simulink model "Model"  (R2021b)
settings: Solver=VariableStepAuto  StartTime=0.0  StopTime=SimTime  FixedStep=1  RelTol=1e-13  AbsTol=1e-13
values from neighbouring files (symbols this model uses):
  a = (39376)*1e3    (= 39376000)    [ScriptGroup20.m]
  alphaxy = (alphaxy/3)^2    (= 2.60887104e-10)    [ScriptGroup20.m]
  alphaz = (alphaz/3)^2    (= 3.75687767111e-08)    [ScriptGroup20.m]
  Aorthsens = 1e-3.*[1000,0.2,0.2;0.2,1000,0.2;0.2,0.2,1000]    [ScriptGroup20.m]
  burn_angle = deg2rad(30)    [ScriptGroup20.m]
  Controlled = 1    [ScriptGroup20.m]
  e = 0.7596    [ScriptGroup20.m]
  fgyro = 5    [ScriptGroup20.m]
  Fmax = 0.325/2    (= 0.1625)    [ScriptGroup20.m]
  fst = 5    [ScriptGroup20.m]
  hr0 = hrwslew(:,end)    [ScriptGroup20.m]
  i = deg2rad(28.4252)    [ScriptGroup20.m]
  I_tensor = I_unpacked    [ScriptGroup20.m]
  Iinv_tensor = inv(I_tensor)    [ScriptGroup20.m]
  Kdtrack = Kdtrack_track    (= 0.009)    [ScriptGroup20.m]
  Kpdet = 0.3    [ScriptGroup20.m]
  Kptrack = Kptrack_track    (= 0.009)    [ScriptGroup20.m]
  m_sc = factor*[1;1;1]    [ScriptGroup20.m]
  maxH = 50*1e-3    (= 0.05)    [ScriptGroup20.m]
  maxT = 8*1e-3    (= 0.008)    [ScriptGroup20.m]
  ModCont = 1    [ScriptGroup20.m]
  mu = 3.98600433e+5*1e9    (= 398600433000000)    [ScriptGroup20.m]
  normals = [n1,n2,n3,n4,n5,n6,n7,n8,n9,n10]    [ScriptGroup20.m]
  omega = deg2rad(0)    [ScriptGroup20.m]
  phi0 = Angtrueslew(1,1,end)    [ScriptGroup20.m]
  propmat = [rhos_sc;rhod_sc;rhos_sp;rhod_sp]    [ScriptGroup20.m]
  propsurf = [A1,A2,A3,A1,A2,A3,A7,A7,A9,A9]    [ScriptGroup20.m]
  psi0 = Angtrueslew(3,1,end)    [ScriptGroup20.m]
  r_cpTocm = [r1,r2,r3,r4,r5,r6,r7,r8,r9,r10]-ones(3,10).*cm    [ScriptGroup20.m]
  Re = 6371.01*1e3    (= 6371010)    [ScriptGroup20.m]
  sigma = deg2rad(0)    [ScriptGroup20.m]
  starcat = zeros(height(starcattab)-2,2)    [ScriptGroup20.m]
  T = R2*R1*[x*sin(gamma),-x*sin(gamma),x*sin(gamma),-x*sin(gamma);         -x*cos(gamma),l*sin(gamma),x*cos(gamma),-l*sin(gamma);         -l*sin(gamma),x*cos(gamma),l*sin(gamma),-x*cos(gamma)]    [ScriptGroup20.m]
  theta0 = Angtrueslew(2,1,end)    [ScriptGroup20.m]
  theta0orb = forbitslew(end)    [ScriptGroup20.m]
  thetb = thetb^2    [ScriptGroup20.m]
  thetn = thetn^2    [ScriptGroup20.m]
  thetsperc = 5*1e-4    (= 0.0005)    [ScriptGroup20.m]
  w = null(T)    [ScriptGroup20.m]
  w0_vector = wgyroslew(:,1,end)    [ScriptGroup20.m]
  w_lim = deg2rad(3)    [ScriptGroup20.m]
undefined symbols (not defined in the file or in its folder): DiscIntNeverNeededParam, phi_0, psi_0, theta_0
libraries: dspindex x22, matrix_library x20, vrlib x6, dspinverses x3, simulink_extras x3, dspfdesign x3, dspmtrx3 x2, simulink x1
(part 1 of 2)
settings Model: Creator=giova  LastModifiedBy=giova
settings SolverCC: ZeroCrossAlgorithm=Adaptive
settings OptimizationCC: BlockReduction=off  DefaultParameterBehavior=Inlined  BufferReuse=off
settings DebuggingCC: IgnoredZcDiagnostic=none

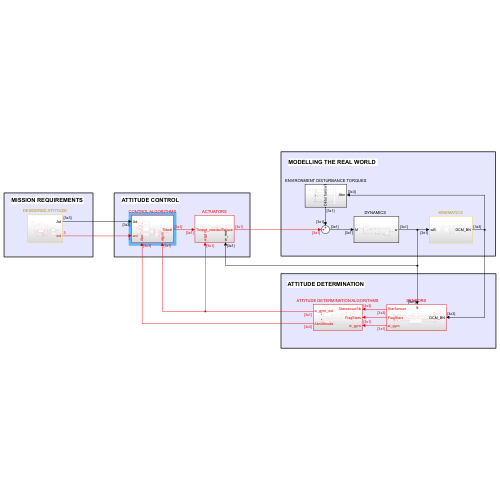
[thumbnail: Simulink's stored preview of the top-level diagram]
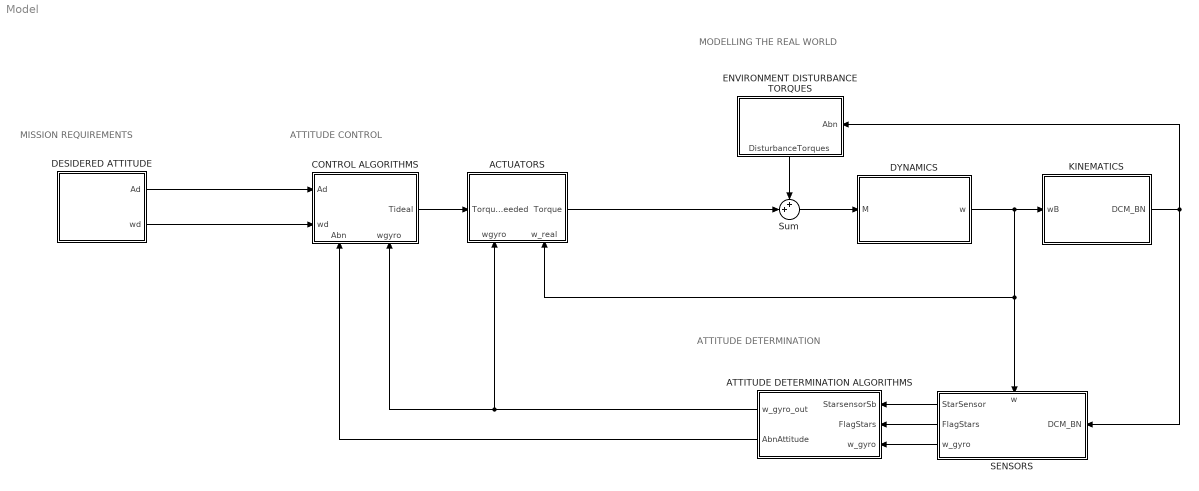
== system Model ==
  note: MODELLING THE REAL WORLD
  note: ATTITUDE DETERMINATION
  note: MISSION REQUIREMENTS
  note: ATTITUDE CONTROL
  ACTUATORS : Subsystem
      settings: PortSchema="{\"entries\":[{\"content\":{\"sides\":[{\"content\":{\"connectorIds\":[\"In1\"]},\"type\":\"ConnectorPlacement.EquallySpacedRectSide\",\"uuid\":\"28bcfce0-0d34-469d-9776-74cc58e318fa\"},{\"content\":{\"connectorIds\":[\"Out1\"],\"side\":\"RIGHT\"},\"type\":\"ConnectorPlacement.EquallySpacedRectSide\",\"uuid\":\"2255c173-df7a-4664-85cc-96c785adaea5\"},{\"content\":{\"connectorIds\":[],\"side\":\"TOP\"},\"type\":\"ConnectorPlacement.EquallySpacedRectSide\",\"uuid\":\"32c912d7-9334-4d54-9f32-8ee23b9abac0\"},{\"content\":{\"connectorIds\":[\"In2\",\"In3\"],\"side\":\"BOTTOM\"},\"type\":\"ConnectorPlacement.EquallySpacedRectSide\",\"uuid\":\"2cb89a57-816b-4867-95bb-5d60911795f4\"}]},\"type\":\"ConnectorPlacement.EquallySpacedConnector\",\"uuid\":\"77867389-a468-4a3c-acb5-d08783c7db16\"}],\"packageUris\":[\"http://schema.mathworks.com/mf0/Connector/R2020b\"],\"version\":\"1.0\"}"
  ATTITUDE DETERMINATION ALGORITHMS : Subsystem
  CONTROL ALGORITHMS : Subsystem
      settings: PortSchema="{\"entries\":[{\"content\":{\"sides\":[{\"content\":{\"connectorIds\":[\"In1\",\"In2\"]},\"type\":\"ConnectorPlacement.EquallySpacedRectSide\",\"uuid\":\"73dddf99-4801-43df-975c-c163be84342b\"},{\"content\":{\"connectorIds\":[\"Out1\"],\"side\":\"RIGHT\"},\"type\":\"ConnectorPlacement.EquallySpacedRectSide\",\"uuid\":\"0da970fe-52f5-407f-b1e9-9d4b0160e11a\"},{\"content\":{\"connectorIds\":[],\"side\":\"TOP\"},\"type\":\"ConnectorPlacement.EquallySpacedRectSide\",\"uuid\":\"7ba04c9a-5ad7-470a-a631-d233976ad8b8\"},{\"content\":{\"connectorIds\":[\"In3\",\"In4\"],\"side\":\"BOTTOM\"},\"type\":\"ConnectorPlacement.EquallySpacedRectSide\",\"uuid\":\"5f2d3d06-e891-478c-9602-3776d7c735db\"}]},\"type\":\"ConnectorPlacement.EquallySpacedConnector\",\"uuid\":\"a8e1a751-f603-45b5-97f1-265969e24c76\"}],\"packageUris\":[\"http://schema.mathworks.com/mf0/Connector/R2020b\"],\"version\":\"1.0\"}"
  DESIDERED ATTITUDE : Subsystem
  "DYNAMICS  " : Subsystem
  ENVIRONMENT DISTURBANCE TORQUES : Subsystem
      settings: PortSchema="{\"entries\":[{\"content\":{\"sides\":[{\"content\":{\"connectorIds\":[\"In1\"]},\"type\":\"ConnectorPlacement.EquallySpacedRectSide\",\"uuid\":\"a2be9383-99de-4e0f-aff6-078514624980\"},{\"content\":{\"connectorIds\":[],\"side\":\"RIGHT\"},\"type\":\"ConnectorPlacement.EquallySpacedRectSide\",\"uuid\":\"8c8f0942-4a2a-4cb8-b252-92284a086b4d\"},{\"content\":{\"connectorIds\":[\"Out1\"],\"side\":\"TOP\"},\"type\":\"ConnectorPlacement.EquallySpacedRectSide\",\"uuid\":\"b1ad7016-209b-4a42-9402-dc7624b55aba\"}]},\"type\":\"ConnectorPlacement.EquallySpacedConnector\",\"uuid\":\"7a786cca-b338-4110-b1b1-81221cfdfe5d\"}],\"packageUris\":[\"http://schema.mathworks.com/mf0/Connector/R2020b\"],\"version\":\"1.0\"}"
  KINEMATICS : Subsystem
  SENSORS : Subsystem
      settings: PortSchema="{\"entries\":[{\"content\":{\"sides\":[{\"content\":{\"connectorIds\":[\"In1\"]},\"type\":\"ConnectorPlacement.EquallySpacedRectSide\",\"uuid\":\"b510f6ef-f21e-411c-8ea4-8a9ce0e96801\"},{\"content\":{\"connectorIds\":[\"Out1\",\"Out2\",\"Out3\"],\"side\":\"RIGHT\"},\"type\":\"ConnectorPlacement.EquallySpacedRectSide\",\"uuid\":\"2c17a393-d83e-490b-b8d9-3edd4b192ceb\"},{\"content\":{\"connectorIds\":[],\"side\":\"TOP\"},\"type\":\"ConnectorPlacement.EquallySpacedRectSide\",\"uuid\":\"72c4e30b-e03c-45bc-abfe-ce46fe4af89d\"},{\"content\":{\"connectorIds\":[\"In2\"],\"side\":\"BOTTOM\"},\"type\":\"ConnectorPlacement.EquallySpacedRectSide\",\"uuid\":\"41e20ae9-4ca7-4038-b613-5a3bc8a297c6\"}]},\"type\":\"ConnectorPlacement.EquallySpacedConnector\",\"uuid\":\"248ff9f1-2acb-4da2-b04a-a2681fb74a40\"}],\"packageUris\":[\"http://schema.mathworks.com/mf0/Connector/R2020b\"],\"version\":\"1.0\"}"
  Sum : Sum  Inputs=++|
  wires:
  KINEMATICS/1(DCM_BN) -> SENSORS/1(DCM_BN), ENVIRONMENT DISTURBANCE TORQUES/1(Abn)
  "DYNAMICS  "/1(w) -> KINEMATICS/1(wB), ACTUATORS/3(w_real), SENSORS/2(w)
  Sum/1 -> "DYNAMICS  "/1(M)
  ENVIRONMENT DISTURBANCE TORQUES/1(DisturbanceTorques) -> Sum/1
  SENSORS/2(FlagStars) -> ATTITUDE DETERMINATION ALGORITHMS/2(FlagStars)
  SENSORS/3(StarSensor) -> ATTITUDE DETERMINATION ALGORITHMS/1(StarsensorSb)
  SENSORS/1(w_gyro) -> ATTITUDE DETERMINATION ALGORITHMS/3(w_gyro)
  ACTUATORS/1(Torque) -> Sum/2
  DESIDERED ATTITUDE/1(Ad) -> CONTROL ALGORITHMS/1(Ad)
  ATTITUDE DETERMINATION ALGORITHMS/1(w_gyro_out) -> CONTROL ALGORITHMS/4(wgyro), ACTUATORS/2(wgyro)
  ATTITUDE DETERMINATION ALGORITHMS/2(AbnAttitude) -> CONTROL ALGORITHMS/3(Abn)
  CONTROL ALGORITHMS/1(Tideal) -> ACTUATORS/1(Torque_needed)
  DESIDERED ATTITUDE/2(wd) -> CONTROL ALGORITHMS/2(wd)

== system Model/ACTUATORS ==
  Torque_needed : Inport
  wgyro : Inport  Port=2
  w_real : Inport  Port=3
  Constant : Constant  Value=[0;0;0]
  RW : Subsystem
  Sum : Sum
  Switch : Switch  Criteria=u2 > Threshold
  Thruster : Subsystem
  To Workspace : ToWorkspace  VariableName=simout7  SaveFormat=Timeseries  SampleTime=-1
  To Workspace1 : ToWorkspace  VariableName=simout9  SaveFormat=Timeseries  SampleTime=-1
  Torque : Outport
  wires:
  Sum/1 -> To Workspace/1, Torque/1
  wgyro/1 -> RW/2(wgyro)
  RW/2(Treal) -> Sum/2
  Thruster/1(TorqueReal) -> Switch/1
  Constant/1 -> Switch/3
  Switch/1 -> To Workspace1/1, Sum/1
  Torque_needed/1 -> RW/1(Torque_needed), Thruster/1(Torqueneeded)
  RW/1(FlagDesat) -> Switch/2
  w_real/1 -> RW/3(w_real)

== system Model/ATTITUDE DETERMINATION ALGORITHMS ==
  StarsensorSb : Inport
  FlagStars : Inport  Port=2
  w_gyro : Inport  Port=3
  Kinematics with update from Star Tracker1 : Subsystem
  Switch : Switch  Criteria=u2 ~= 0
  SwitchAttitudeDetermination : Subsystem
  To Workspace : ToWorkspace  VariableName=simout1  SaveFormat=Timeseries  SampleTime=-1
  w_gyro_out : Outport
  AbnAttitude : Outport  Port=2
  wires:
  Kinematics with update from Star Tracker1/1(DCM_BN_gyro) -> Switch/3
  SwitchAttitudeDetermination/1(star_out) -> Kinematics with update from Star Tracker1/3(star_out), Switch/2
  FlagStars/1 -> SwitchAttitudeDetermination/2(FlagStars)
  StarsensorSb/1 -> Switch/1, Kinematics with update from Star Tracker1/1(DCM_BN_star)
  Switch/1 -> AbnAttitude/1, To Workspace/1, SwitchAttitudeDetermination/3(Abnsensors)
  w_gyro/1 -> SwitchAttitudeDetermination/1(wB_m), w_gyro_out/1, Kinematics with update from Star Tracker1/2(wB_m)

== system Model/CONTROL ALGORITHMS ==
  Ad : Inport
  wd : Inport  Port=2
  Abn : Inport  Port=3
  wgyro : Inport  Port=4
  Constant : Constant  Value=ModCont
  Constant1 : Constant  Value=[0;0;0]
  Constant2 : Constant  Value=Controlled
  De-tumbling : Subsystem
  Pointing error : Subsystem
      settings: PortSchema="{\"entries\":[{\"content\":{\"sides\":[{\"content\":{\"connectorIds\":[]},\"type\":\"ConnectorPlacement.EquallySpacedRectSide\",\"uuid\":\"59077e71-7c09-4a90-bf3b-715fb2f3e64a\"},{\"content\":{\"connectorIds\":[\"In1\",\"In2\"],\"side\":\"RIGHT\"},\"type\":\"ConnectorPlacement.EquallySpacedRectSide\",\"uuid\":\"5359064d-45c1-447c-a242-520af2c8ee16\"},{\"content\":{\"connectorIds\":[],\"side\":\"TOP\"},\"type\":\"ConnectorPlacement.EquallySpacedRectSide\",\"uuid\":\"50cd8bf9-1849-445b-b3a9-8b2cd9485115\"}]},\"type\":\"ConnectorPlacement.EquallySpacedConnector\",\"uuid\":\"6167e8e7-e0c2-4106-8eb9-df9ff1faf5b0\"}],\"packageUris\":[\"http://schema.mathworks.com/mf0/Connector/R2020b\"],\"version\":\"1.0\"}"
  Switch : Switch  Criteria=u2 > Threshold
  Switch1 : Switch  Criteria=u2 > Threshold
  Tracking : Subsystem
  Tideal : Outport
  wires:
  Abn/1 -> Tracking/2(Abn), Pointing error/2(Abnsen)
  Ad/1 -> Tracking/1(Ad), Pointing error/1(Ad)
  wgyro/1 -> Tracking/4(wgyro), De-tumbling/1(w)
  De-tumbling/1(Tdet) -> Switch/3
  Constant/1 -> Switch/2
  Constant1/1 -> Switch1/3
  Constant2/1 -> Switch1/2
  Tracking/1(Ttrack) -> Switch/1
  Switch/1 -> Switch1/1
  Switch1/1 -> Tideal/1
  wd/1 -> Tracking/3(wd)

== system Model/DESIDERED ATTITUDE ==
  Constant : Constant  Value=sigma
  Constant1 : Constant  Value=i
  Constant2 : Constant  Value=omega
  Constant3 : Constant  Value=a
  Constant4 : Constant  Value=e
  Constant5 : Constant  Value=0
  Discrete-Time Integrator : DiscreteIntegrator  InitialCondition=theta0orb  SampleTime=-1  ICPrevOutput=DiscIntNeverNeededParam  ICPrevScaledInput=DiscIntNeverNeededParam
  From N to eph : MATLAB Function  TreatAsAtomicUnit=on
  From eph to rthetah : MATLAB Function  TreatAsAtomicUnit=on
  Mux : Mux  Inputs=3
  Subsystem1 : Subsystem
  To Workspace : ToWorkspace  VariableName=simout8  SaveFormat=Timeseries  SampleTime=-1
  Ad : Outport
  wd : Outport  Port=2
  wires:
  Constant/1 -> From N to eph/1(sigma)
  Constant1/1 -> From N to eph/2(i)
  Constant2/1 -> From N to eph/3(omega)
  Discrete-Time Integrator/1 -> To Workspace/1, From eph to rthetah/2(theta), Subsystem1/3(Theta)  "theta"
  Constant4/1 -> Subsystem1/1(e)
  Constant3/1 -> Subsystem1/2(a)
  From N to eph/1(Aeph) -> From eph to rthetah/1(Aeph)
  From eph to rthetah/1(Arthetah) -> Ad/1
  Subsystem1/1(ThetaDot) -> Mux/3, Discrete-Time Integrator/1
  Constant5/1 -> Mux/1, Mux/2
  Mux/1 -> wd/1

== system Model/DYNAMICS   ==
  M : Inport
  Constant : Constant  Value=I_tensor
  Constant1 : Constant  Value=Iinv_tensor
  Cross Product : vrlib/Utilities/Cross Product
  Integrator : Integrator  InitialCondition=w0_vector
  Product : Product  Multiplication=Matrix(*)
  Product1 : Product  Multiplication=Matrix(*)
  Sum : Sum  Inputs=+-
  w : Outport
  wires:
  Constant1/1 -> Product1/1
  Sum/1 -> Product1/2  "w'"
  Product1/1 -> Integrator/1
  Cross Product/1 -> Sum/2
  M/1 -> Sum/1
  Constant/1 -> Product/1
  Product/1 -> Cross Product/2
  Integrator/1 -> w/1, Product/2, Cross Product/1  "w"

== system Model/ENVIRONMENT DISTURBANCE TORQUES ==
  Abn : Inport
  Gravity Gradient Torque : Subsystem
  MagneticTorque : Subsystem
  OrbitRadialDirection : Subsystem
  Product1 : Product  Multiplication=Matrix(*)
  SRPTorque : Subsystem
  Subsystem : Subsystem
  Sum : Sum  Inputs=+++
  SunPositionRespectN : Subsystem
  To Workspace : ToWorkspace  VariableName=simout6  SaveFormat=Timeseries  SampleTime=-1
  DisturbanceTorques : Outport
  wires:
  Sum/1 -> To Workspace/1, DisturbanceTorques/1
  Gravity Gradient Torque/1(GravityTorque) -> Sum/3
  OrbitRadialDirection/2(Aln) -> Gravity Gradient Torque/2(Aln)
  MagneticTorque/1(MagneticTorque) -> Sum/1
  SunPositionRespectN/1(sn) -> Subsystem/2(rs), Product1/2
  Product1/1 -> SRPTorque/2(sb)  "sb"
  OrbitRadialDirection/1(rn) -> Gravity Gradient Torque/3(rn), Subsystem/1(rn), MagneticTorque/1(rn)
  SRPTorque/1(SRPTorque) -> Sum/2
  Abn/1 -> MagneticTorque/2(Abn), Product1/1, Gravity Gradient Torque/1(Abn)
  Subsystem/1(flag_eclipse) -> SRPTorque/1(SwitchEclipse)

== system Model/KINEMATICS ==
  wB : Inport
  312 Euler Angles : Subsystem
  313 Euler Angles : Subsystem
  Constant : Constant  Value=[phi0;theta0;psi0]
  Delay One Step : Delay  DelayLength=1  InitialConditionSource=Input port
      settings: InputPortMap=u0,p4
  Delay One Step1 : Delay  DelayLength=1  InitialConditionSource=Input port
      settings: InputPortMap=u0,p4
  Factotum Switch : MATLAB Function  TreatAsAtomicUnit=on
  FinalConditions : Subsystem
  Initial condition : MATLAB Function  TreatAsAtomicUnit=on
  Switch : Switch  Criteria=u2 ~= 0
  DCM_BN : Outport
  wires:
  wB/1 -> 313 Euler Angles/1(wB), 312 Euler Angles/3(wB)
  312 Euler Angles/1(DCM_BN_312) -> Switch/1
  313 Euler Angles/1(DCM_BN_313) -> Switch/3
  Factotum Switch/1(IC_312) -> 312 Euler Angles/1(IC_312)
  Factotum Switch/3(IC_313) -> 313 Euler Angles/3(IC_313)
  Switch/1 -> DCM_BN/1, FinalConditions/1(DCM), Delay One Step1/1
  Factotum Switch/2(flagOut) -> Delay One Step/1, 313 Euler Angles/2(flag), Switch/2, 312 Euler Angles/2(flag)
  Delay One Step/1 -> Factotum Switch/2(flagIn)
  Delay One Step1/1 -> Factotum Switch/1(DCM_BN)
  Constant/1 -> Initial condition/1(EA_BN_0)
  Initial condition/2(flagIn_0) -> Delay One Step/2
  Initial condition/1(DCM_BN_0) -> Delay One Step1/2

== system Model/SENSORS ==
  DCM_BN : Inport
  w : Inport  Port=2
  Gyro : Subsystem
  StarCat : Subsystem
  To Workspace : ToWorkspace  VariableName=simout  SaveFormat=Timeseries  SampleTime=-1
  Zero-Order Hold1 : ZeroOrderHold  SampleTime=1/fst
  Zero-Order Hold2 : ZeroOrderHold  SampleTime=1/fst
  w_gyro : Outport
  FlagStars : Outport  Port=2
  StarSensor : Outport  Port=3
  wires:
  DCM_BN/1 -> Zero-Order Hold1/1
  Zero-Order Hold1/1 -> StarCat/1(Abn)
  w/1 -> Zero-Order Hold2/1
  Zero-Order Hold2/1 -> Gyro/1(w)
  Gyro/1(w_gyro) -> To Workspace/1, w_gyro/1
  StarCat/1(StarSensor) -> StarSensor/1
  StarCat/2(FlagStars) -> FlagStars/1

== system Model/ACTUATORS/RW ==
  Torque_needed : Inport
  wgyro : Inport  Port=2
  w_real : Inport  Port=3
  Aconfiguration : Constant  Value=[1,0,0,1/sqrt(3);0,1,0,1/sqrt(3);0,0,1,1/sqrt(3)]  SampleTime=1/fgyro
  Mapping actuator : Subsystem
  RealRW : Subsystem
      settings: PortSchema="{\"entries\":[{\"content\":{\"sides\":[{\"content\":{\"connectorIds\":[\"In1\",\"In2\"]},\"type\":\"ConnectorPlacement.EquallySpacedRectSide\",\"uuid\":\"4cf3556b-d79b-4b35-83c7-165ec12fb347\"},{\"content\":{\"connectorIds\":[\"Out1\",\"Out2\"],\"side\":\"RIGHT\"},\"type\":\"ConnectorPlacement.EquallySpacedRectSide\",\"uuid\":\"b017f686-de2a-46f5-bc21-38e4657d98f2\"},{\"content\":{\"connectorIds\":[\"In3\"],\"side\":\"TOP\"},\"type\":\"ConnectorPlacement.EquallySpacedRectSide\",\"uuid\":\"e19596cf-63b5-4569-a83e-a83db9975230\"}]},\"type\":\"ConnectorPlacement.EquallySpacedConnector\",\"uuid\":\"677db8a5-061d-4d8b-93d2-fe0edb0a0b58\"}],\"packageUris\":[\"http://schema.mathworks.com/mf0/Connector/R2020b\"],\"version\":\"1.0\"}"
  FlagDesat : Outport
  Treal : Outport  Port=2
  wires:
  Torque_needed/1 -> Mapping actuator/1(Uideal)
  wgyro/1 -> Mapping actuator/2(w_gyro)
  Aconfiguration/1 -> RealRW/1(Configuration), Mapping actuator/3(Configuration)
  RealRW/1(Ureal) -> Treal/1
  Mapping actuator/1(ElectricMotor) -> RealRW/3(Mr)
  RealRW/2(FlagDesat) -> FlagDesat/1
  w_real/1 -> RealRW/2(w_real)

== system Model/ACTUATORS/Thruster ==
  Torqueneeded : Inport
  Constant : Constant  Value=T  SampleTime=1/fgyro
  Constant4 : Constant  Value=w
  Divide : Product  Inputs=*/
  Max : MinMax  Function=max
  On/Off logic : Subsystem
  Product : Product  Multiplication=Matrix(*)
  Product1 : Product
  Product2 : Product  Multiplication=Matrix(*)
  Pseudoinverse : dspinverses/Pseudoinverse  wanterr=off  SimulateUsing=Interpreted execution
      settings: SourceProductBaseCode=DS
  Scope : Scope
  Sum : Sum
  TorqueReal : Outport
  wires:
  Constant/1 -> Pseudoinverse/1, Product2/1
  Torqueneeded/1 -> Product/2
  Pseudoinverse/1 -> Product/1
  Product/1 -> Sum/2, Divide/1
  Divide/1 -> Max/1
  Product1/1 -> Sum/1
  Constant4/1 -> Product1/2, Divide/2  "null space"
  Product2/1 -> TorqueReal/1
  On/Off logic/1(Freal) -> Product2/2, Scope/1
  Sum/1 -> On/Off logic/1(Fideal)
  Max/1 -> Product1/1

== system Model/ATTITUDE DETERMINATION ALGORITHMS/Kinematics with update from Star Tracker1 ==
  DCM_BN_star : Inport
  wB_m : Inport  Port=2
  star_out : Inport  Port=3
  312 Euler Angles : Subsystem
  313 Euler Angles : Subsystem
  Delay One Step : Delay  DelayLength=1  InitialConditionSource=Input port
      settings: InputPortMap=u0,p4
  Delay One Step1 : Delay  DelayLength=1  InitialConditionSource=Input port
      settings: InputPortMap=u0,p4
  Factotum Switch : MATLAB Function  TreatAsAtomicUnit=on
  Initial condition : MATLAB Function  TreatAsAtomicUnit=on
  MATLAB Function : MATLAB Function  TreatAsAtomicUnit=on
  MATLAB Function1 : MATLAB Function  TreatAsAtomicUnit=on
  Scope : Scope
  Switch : Switch  Criteria=u2 ~= 0
  DCM_BN_gyro : Outport
  wires:
  Factotum Switch/1(IC_312) -> MATLAB Function/2(IC_312_in)
  Factotum Switch/3(IC_313) -> MATLAB Function1/3(IC_313_in)
  MATLAB Function1/2(IC_313_out) -> 313 Euler Angles/3(IC_313)
  MATLAB Function1/1(flag_out) -> 313 Euler Angles/2(flag)
  star_out/1 -> MATLAB Function1/1(star_out), MATLAB Function/4(star_out)
  MATLAB Function/2(flag_out) -> 312 Euler Angles/2(flag)
  MATLAB Function/1(IC_312_out) -> 312 Euler Angles/1(IC_312)
  Initial condition/1(flagIn_0) -> Delay One Step/2
  DCM_BN_star/1 -> MATLAB Function/1(DCM_BN_star), Delay One Step1/2, MATLAB Function1/4(DCM_BN_star), Initial condition/1(DCM_BN_star)
  Delay One Step1/1 -> Factotum Switch/1(DCM_BN)
  Delay One Step/1 -> Factotum Switch/2(flagIn)
  Factotum Switch/2(flagOut) -> Scope/1, Switch/2, Delay One Step/1, MATLAB Function1/2(flag_in), MATLAB Function/3(flag_in)
  Switch/1 -> Delay One Step1/1, DCM_BN_gyro/1
  313 Euler Angles/1(DCM_BN_313) -> Switch/3
  312 Euler Angles/1(DCM_BN_312) -> Switch/1
  wB_m/1 -> 312 Euler Angles/3(wB), 313 Euler Angles/1(wB)

== system Model/ATTITUDE DETERMINATION ALGORITHMS/SwitchAttitudeDetermination ==
  wB_m : Inport
  FlagStars : Inport  Port=2
  Abnsensors : Inport  Port=3
  Constant : Constant  Value=[0; 0; 1]  VectorParams1D=off
  Constant1 : Constant  Value=burn_angle
  Constant2 : Constant  Value=w_lim
  Delay : Delay  DelayLength=1  InitialCondition=[1,0,0;0,1,0;0,0,1]
  Dot Product : DotProduct  InputSameDT=on  OutDataTypeStr=Inherit: Inherit via internal rule
  MATLAB Function : MATLAB Function  TreatAsAtomicUnit=on
  Product : Product  Multiplication=Matrix(*)
  SunPositionRespectN : Subsystem
  star_out : Outport
  wires:
  SunPositionRespectN/1(sn) -> Product/2
  Constant2/1 -> MATLAB Function/4(w_lim)
  Constant1/1 -> MATLAB Function/3(burn_angle)
  Constant/1 -> Dot Product/2
  FlagStars/1 -> MATLAB Function/5(FlagStars)
  Abnsensors/1 -> Delay/1
  Dot Product/1 -> MATLAB Function/2(cos_alpha)
  wB_m/1 -> MATLAB Function/1(wB_m)
  MATLAB Function/1(star_out) -> star_out/1
  Product/1 -> Dot Product/1
  Delay/1 -> Product/1

== system Model/CONTROL ALGORITHMS/De-tumbling ==
  w : Inport
  Gain : Gain  Gain=-Kpdet
  Tdet : Outport
  wires:
  w/1 -> Gain/1
  Gain/1 -> Tdet/1

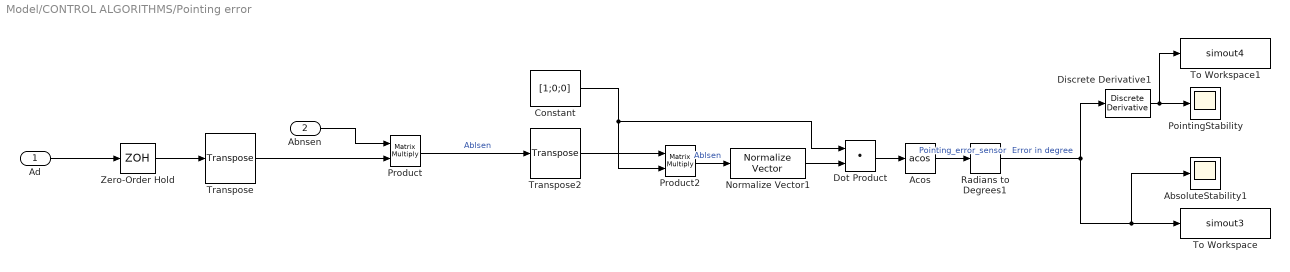
== system Model/CONTROL ALGORITHMS/Pointing error ==
  Ad : Inport
  Abnsen : Inport  Port=2
  AbsoluteStability1 : Scope
  Acos : Trigonometry  Operator=acos
  Constant : Constant  Value=[1;0;0]
  Discrete Derivative1 : simulink/Discrete/Discrete Derivative  gainval=1.0  ICPrevScaledInput=0.0  OutMin=[]  OutMax=[]  OutDataType=fixdt(1, 16)  OutScaling=2^-10  DoSatur=off
  Dot Product : DotProduct  InputSameDT=on  OutDataTypeStr=Inherit: Inherit via internal rule
  Normalize Vector1 : vrlib/Utilities/Normalize Vector  maxzero=0
  PointingStability : Scope
  Product : Product  Multiplication=Matrix(*)
  Product2 : Product  Multiplication=Matrix(*)
  Radians to Degrees1 : simulink_extras/Transformations/Radians to Degrees
  To Workspace : ToWorkspace  VariableName=simout3  SaveFormat=Timeseries  SampleTime=-1
  To Workspace1 : ToWorkspace  VariableName=simout4  SaveFormat=Timeseries  SampleTime=-1
  Transpose : matrix_library/Transpose
      settings: SourceProductBaseCode=SL
  Transpose2 : matrix_library/Transpose
      settings: SourceProductBaseCode=SL
  Zero-Order Hold : ZeroOrderHold  SampleTime=1/fgyro
  wires:
  Ad/1 -> Zero-Order Hold/1
  Zero-Order Hold/1 -> Transpose/1
  Product/1 -> Transpose2/1  "Ablsen"
  Transpose/1 -> Product/2
  Abnsen/1 -> Product/1
  Transpose2/1 -> Product2/1
  Constant/1 -> Dot Product/1, Product2/2
  Product2/1 -> Normalize Vector1/1  "Ablsen"
  Dot Product/1 -> Acos/1
  Acos/1 -> Radians to Degrees1/1  "Pointing_error_sensor"
  Discrete Derivative1/1 -> To Workspace1/1, PointingStability/1
  Radians to Degrees1/1 -> Discrete Derivative1/1, To Workspace/1, AbsoluteStability1/1  "Error in degree"
  Normalize Vector1/1 -> Dot Product/2

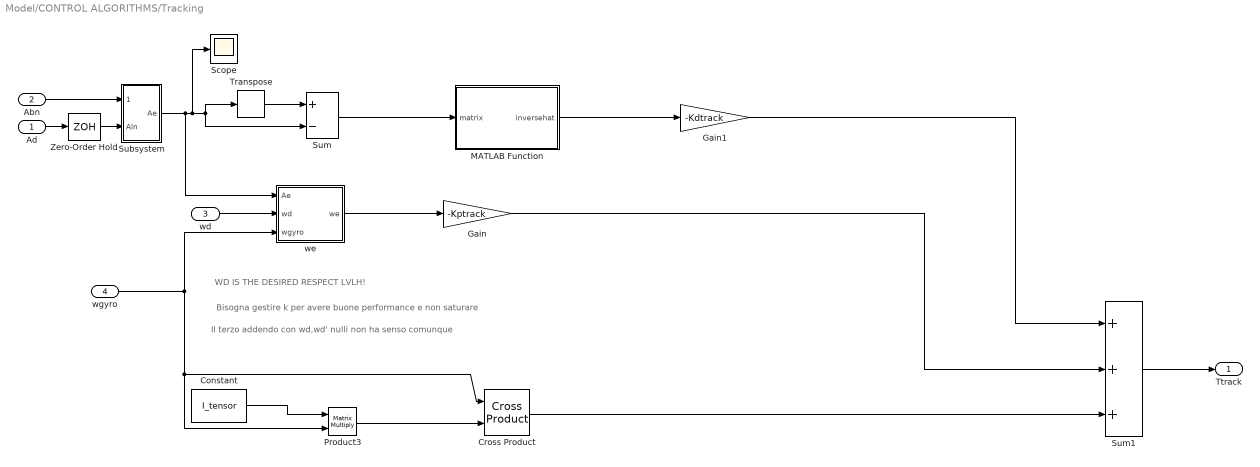
== system Model/CONTROL ALGORITHMS/Tracking ==
  note: Il terzo addendo con wd,wd' nulli non ha senso comunque
  note: Bisogna gestire k per avere buone performance e non saturare
  note: WD IS THE DESIRED RESPECT LVLH!
  Ad : Inport
  Abn : Inport  Port=2
  wd : Inport  Port=3
  wgyro : Inport  Port=4
  Constant : Constant  Value=I_tensor
  Cross Product : matrix_library/Cross Product
      settings: SourceProductBaseCode=SL
  Gain : Gain  Gain=-Kptrack
  Gain1 : Gain  Gain=-Kdtrack
  MATLAB Function : MATLAB Function  TreatAsAtomicUnit=on
  Product3 : Product  Multiplication=Matrix(*)
  Scope : Scope
  Subsystem : Subsystem
  Sum : Sum  Inputs=+-
  Sum1 : Sum  Inputs=+++
  Transpose : matrix_library/Transpose
      settings: SourceProductBaseCode=SL
  Zero-Order Hold : ZeroOrderHold  SampleTime=-1
  we : Subsystem
  Ttrack : Outport
  wires:
  Sum1/1 -> Ttrack/1
  Transpose/1 -> Sum/1
  Subsystem/1(Ae) -> we/1(Ae), Scope/1, Transpose/1, Sum/2
  Constant/1 -> Product3/1
  Product3/1 -> Cross Product/2
  Cross Product/1 -> Sum1/3
  wgyro/1 -> we/3(wgyro), Product3/2, Cross Product/1
  Gain/1 -> Sum1/2
  Sum/1 -> MATLAB Function/1(matrix)
  MATLAB Function/1(inversehat) -> Gain1/1
  we/1(we) -> Gain/1
  Ad/1 -> Zero-Order Hold/1
  Gain1/1 -> Sum1/1
  Zero-Order Hold/1 -> Subsystem/2(Aln)
  Abn/1 -> Subsystem/1(Abn)
  wd/1 -> we/2(wd)

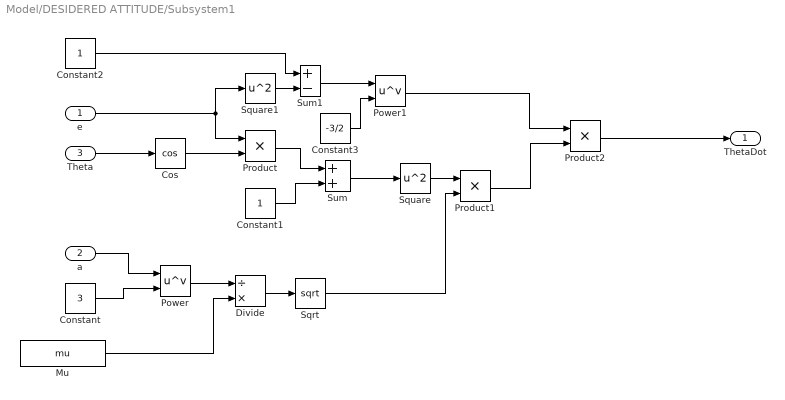
== system Model/DESIDERED ATTITUDE/Subsystem1 ==
  e : Inport
  a : Inport  Port=2
  Theta : Inport  Port=3
  Constant : Constant  Value=3
  Constant1 : Constant
  Constant2 : Constant
  Constant3 : Constant  Value=-3/2
  Cos : Trigonometry  Operator=cos
  Divide : Product  Inputs=/*
  Mu : Constant  Value=mu
  Power : Math  Operator=pow  SaturateOnIntegerOverflow=on
  Power1 : Math  Operator=pow  SaturateOnIntegerOverflow=on
  Product : Product
  Product1 : Product
  Product2 : Product
  Sqrt : Sqrt  SaturateOnIntegerOverflow=on
  Square : Math  Operator=square  SaturateOnIntegerOverflow=on
  Square1 : Math  Operator=square  SaturateOnIntegerOverflow=on
  Sum : Sum
  Sum1 : Sum  Inputs=+-
  ThetaDot : Outport
  wires:
  Constant/1 -> Power/2
  a/1 -> Power/1
  Power/1 -> Divide/1
  Mu/1 -> Divide/2
  Divide/1 -> Sqrt/1
  Theta/1 -> Cos/1
  Cos/1 -> Product/2
  e/1 -> Product/1, Square1/1
  Constant1/1 -> Sum/2
  Product/1 -> Sum/1
  Sum/1 -> Square/1
  Square/1 -> Product1/1
  Sqrt/1 -> Product1/2
  Square1/1 -> Sum1/2
  Constant2/1 -> Sum1/1
  Sum1/1 -> Power1/1
  Constant3/1 -> Power1/2
  Product1/1 -> Product2/2
  Power1/1 -> Product2/1
  Product2/1 -> ThetaDot/1

== system Model/ENVIRONMENT DISTURBANCE TORQUES/Gravity Gradient Torque ==
  Abn : Inport
  Aln : Inport  Port=2
  rn : Inport  Port=3
  Constant : Constant  Value=[1;0;0]
  Constant1 : Constant  Value=I_tensor
  MATLAB Function : MATLAB Function  TreatAsAtomicUnit=on
  Product : Product  Multiplication=Matrix(*)
  Product1 : Product  Multiplication=Matrix(*)
  Sqrt : Sqrt  SaturateOnIntegerOverflow=on
  Square : Math  Operator=square  SaturateOnIntegerOverflow=on
  Sum of Elements : Sum  Inputs=+
  Transpose : matrix_library/Transpose
      settings: SourceProductBaseCode=SL
  GravityTorque : Outport
  wires:
  Aln/1 -> Transpose/1
  Transpose/1 -> Product/2  "Aln'"
  Abn/1 -> Product/1  "Abn"
  Product/1 -> Product1/1  "Abl"
  Constant/1 -> Product1/2
  MATLAB Function/1(M) -> GravityTorque/1
  Product1/1 -> MATLAB Function/2(c)  "[c1;c2;c3]"
  Constant1/1 -> MATLAB Function/1(I)
  rn/1 -> Square/1
  Sum of Elements/1 -> Sqrt/1
  Square/1 -> Sum of Elements/1
  Sqrt/1 -> MATLAB Function/3(rnorm)

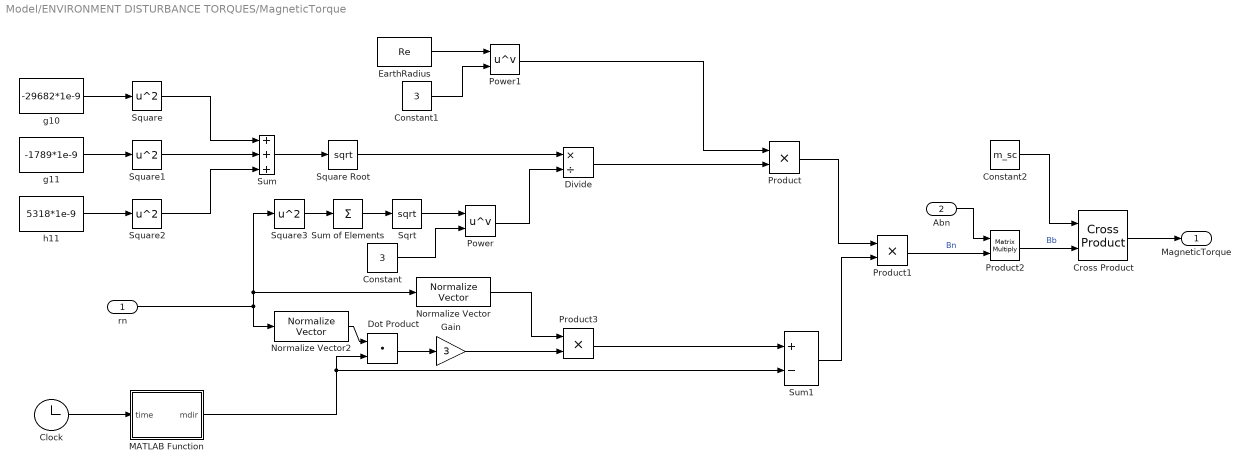
== system Model/ENVIRONMENT DISTURBANCE TORQUES/MagneticTorque ==
  rn : Inport
  Abn : Inport  Port=2
  Clock : Clock
  Constant : Constant  Value=3
  Constant1 : Constant  Value=3
  Constant2 : Constant  Value=m_sc
  Cross Product : matrix_library/Cross Product
      settings: SourceProductBaseCode=SL
  Divide : Product  Inputs=*/
  Dot Product : DotProduct  InputSameDT=on  OutDataTypeStr=Inherit: Inherit via internal rule
  EarthRadius : Constant  Value=Re
  Gain : Gain  Gain=3
  MATLAB Function : MATLAB Function  TreatAsAtomicUnit=on
  Normalize Vector : vrlib/Utilities/Normalize Vector  maxzero=0
  Normalize Vector2 : vrlib/Utilities/Normalize Vector  maxzero=0
  Power : Math  Operator=pow  SaturateOnIntegerOverflow=on
  Power1 : Math  Operator=pow  SaturateOnIntegerOverflow=on
  Product : Product
  Product1 : Product
  Product2 : Product  Multiplication=Matrix(*)
  Product3 : Product
  Sqrt : Sqrt  SaturateOnIntegerOverflow=on
  Square{,1..3} (4 alike) : Math  Operator=square  SaturateOnIntegerOverflow=on
  Square Root : Sqrt  SaturateOnIntegerOverflow=on
  Sum : Sum  Inputs=+++
  Sum of Elements : Sum  Inputs=+
  Sum1 : Sum  Inputs=+-
  g10 : Constant  Value=-29682*1e-9
  g11 : Constant  Value=-1789*1e-9
  h11 : Constant  Value=5318*1e-9
  MagneticTorque : Outport
  wires:
  Clock/1 -> MATLAB Function/1(time)
  g10/1 -> Square/1
  h11/1 -> Square2/1
  g11/1 -> Square1/1
  Square1/1 -> Sum/2
  Square2/1 -> Sum/3
  Square/1 -> Sum/1
  Sum/1 -> Square Root/1
  Square Root/1 -> Divide/1
  Constant/1 -> Power/2
  Power/1 -> Divide/2
  EarthRadius/1 -> Power1/1
  Constant1/1 -> Power1/2
  Divide/1 -> Product/2
  Power1/1 -> Product/1
  Dot Product/1 -> Gain/1
  Product/1 -> Product1/1
  Sum1/1 -> Product1/2
  Product1/1 -> Product2/2  "Bn"
  Abn/1 -> Product2/1
  Cross Product/1 -> MagneticTorque/1
  Square3/1 -> Sum of Elements/1
  Sum of Elements/1 -> Sqrt/1
  Sqrt/1 -> Power/1
  Gain/1 -> Product3/2
  Product3/1 -> Sum1/1
  Product2/1 -> Cross Product/2  "Bb"
  rn/1 -> Normalize Vector2/1, Square3/1, Normalize Vector/1
  MATLAB Function/1(mdir) -> Dot Product/2, Sum1/2
  Normalize Vector/1 -> Product3/1
  Normalize Vector2/1 -> Dot Product/1
  Constant2/1 -> Cross Product/1

== system Model/ENVIRONMENT DISTURBANCE TORQUES/OrbitRadialDirection ==
  Constant : Constant  Value=sigma
  Constant1 : Constant  Value=i
  Constant2 : Constant  Value=omega
  Constant3 : Constant  Value=a
  Constant4 : Constant  Value=e
  Constant5 : Constant  Value=[1;0;0]
  From N to eph : MATLAB Function  TreatAsAtomicUnit=on
  From eph to rthetah : MATLAB Function  TreatAsAtomicUnit=on
  Integrator : Integrator  InitialCondition=theta0orb
  Product : Product
  Product1 : Product  Multiplication=Matrix(*)
  Subsystem : Subsystem
  Subsystem1 : Subsystem
  Transpose : matrix_library/Transpose
      settings: SourceProductBaseCode=SL
  rn : Outport
  Aln : Outport  Port=2
  wires:
  Constant/1 -> From N to eph/1(sigma)
  Constant1/1 -> From N to eph/2(i)
  Constant2/1 -> From N to eph/3(omega)
  Integrator/1 -> From eph to rthetah/2(theta), Subsystem1/3(Theta), Subsystem/1(Theta)  "theta"
  Constant4/1 -> Subsystem1/1(e), Subsystem/2(e)
  Constant3/1 -> Subsystem1/2(a), Subsystem/3(a)
  From N to eph/1(Aeph) -> From eph to rthetah/1(Aeph)
  Constant5/1 -> Product/2
  Subsystem/1(R) -> Product/1
  From eph to rthetah/1(Arthetah) -> Aln/1, Transpose/1
  Product1/1 -> rn/1
  Transpose/1 -> Product1/1
  Product/1 -> Product1/2
  Subsystem1/1(ThetaDot) -> Integrator/1

== system Model/ENVIRONMENT DISTURBANCE TORQUES/SRPTorque ==
  SwitchEclipse : Inport
  sb : Inport  Port=2
  Constant : Constant  Value=propmat
  Constant1 : Constant  Value=propsurf
  Constant2 : Constant  Value=r_cpTocm
  Constant3 : Constant  Value=normals
  Constant4 : Constant  Value=[0;0;0]
  MATLAB Function : MATLAB Function  TreatAsAtomicUnit=on
  Normalize Vector : vrlib/Utilities/Normalize Vector  maxzero=0
  Subsystem : Subsystem
  Switch : Switch  Criteria=u2 > Threshold
  SRPTorque : Outport
  wires:
  Constant/1 -> MATLAB Function/1(propmat)
  Constant1/1 -> MATLAB Function/2(propsurf)
  Constant3/1 -> MATLAB Function/4(normals)
  sb/1 -> Normalize Vector/1
  Normalize Vector/1 -> MATLAB Function/3(sb)
  MATLAB Function/1(Fvec) -> Subsystem/1(Fvec)
  Constant2/1 -> Subsystem/2(r_cpToCM)
  Subsystem/1(Torque) -> Switch/1
  Switch/1 -> SRPTorque/1
  Constant4/1 -> Switch/3
  SwitchEclipse/1 -> Switch/2

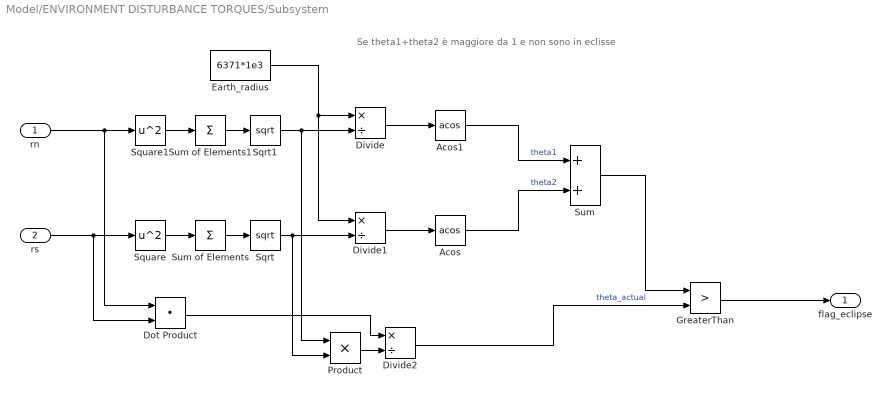
== system Model/ENVIRONMENT DISTURBANCE TORQUES/Subsystem ==
  note: Se theta1+theta2 è maggiore da 1 e non sono in eclisse
  rn : Inport
  rs : Inport  Port=2
  Acos : Trigonometry  Operator=acos
  Acos1 : Trigonometry  Operator=acos
  Divide : Product  Inputs=*/
  Divide1 : Product  Inputs=*/
  Divide2 : Product  Inputs=*/
  Dot Product : DotProduct  InputSameDT=on  OutDataTypeStr=Inherit: Inherit via internal rule
  Earth_radius : Constant  Value=6371*1e3
  GreaterThan : RelationalOperator  Operator=>  OutDataTypeStr=boolean  RndMeth=Simplest
  Product : Product
  Sqrt : Sqrt  SaturateOnIntegerOverflow=on
  Sqrt1 : Sqrt  SaturateOnIntegerOverflow=on
  Square : Math  Operator=square  SaturateOnIntegerOverflow=on
  Square1 : Math  Operator=square  SaturateOnIntegerOverflow=on
  Sum : Sum
  Sum of Elements : Sum  Inputs=+
  Sum of Elements1 : Sum  Inputs=+
  flag_eclipse : Outport
  wires:
  Square/1 -> Sum of Elements/1
  Sum of Elements/1 -> Sqrt/1
  rs/1 -> Dot Product/2, Square/1
  Sum of Elements1/1 -> Sqrt1/1
  Square1/1 -> Sum of Elements1/1
  rn/1 -> Dot Product/1, Square1/1
  Sqrt1/1 -> Product/1, Divide/2
  Sqrt/1 -> Product/2, Divide1/2
  Divide1/1 -> Acos/1
  Divide/1 -> Acos1/1
  Earth_radius/1 -> Divide1/1, Divide/1
  Acos/1 -> Sum/2  "theta2"
  Acos1/1 -> Sum/1  "theta1"
  Product/1 -> Divide2/2
  Dot Product/1 -> Divide2/1
  Sum/1 -> GreaterThan/1
  Divide2/1 -> GreaterThan/2  "theta_actual"
  GreaterThan/1 -> flag_eclipse/1

== system Model/ENVIRONMENT DISTURBANCE TORQUES/SunPositionRespectN ==
  Clock : Clock
  MATLAB Function : MATLAB Function  TreatAsAtomicUnit=on
  Rs : Constant  Value=148390000
  eps : Constant  Value=23.45
  n_sun : Constant  Value=2*pi/31536000
  sn : Outport
  wires:
  eps/1 -> MATLAB Function/1(eps)
  n_sun/1 -> MATLAB Function/2(n_sun)
  Rs/1 -> MATLAB Function/3(Rs)
  Clock/1 -> MATLAB Function/4(time)
  MATLAB Function/1(sn) -> sn/1

== system Model/KINEMATICS/312 Euler Angles ==
  note: Quando il valore del flag
      | sale da 0 a 1 ricomincia
      | ad integrare dalla condizione
      | iniziale che gli sta arrivando
      | in quel momento
  IC_312 : Inport
  flag : Inport  Port=2
  wB : Inport  Port=3
  Create DCM_BN_312 Matrix : MATLAB Function  TreatAsAtomicUnit=on
  Differential Equations 312 : Subsystem
  Integrator : Integrator  ExternalReset=rising  InitialConditionSource=external  InitialCondition=[phi_0; theta_0; psi_0]  WrapState=on
  DCM_BN_312 : Outport
  wires:
  wB/1 -> Differential Equations 312/1(wB)
  Differential Equations 312/1(EA_BN_312_der) -> Integrator/1
  Create DCM_BN_312 Matrix/1(DCM_BN_312) -> DCM_BN_312/1
  Integrator/1 -> Create DCM_BN_312 Matrix/1(EA_BN_312), Differential Equations 312/2(EA_BN_312)
  IC_312/1 -> Integrator/3
  flag/1 -> Integrator/2

== system Model/KINEMATICS/313 Euler Angles ==
  note: Quando il valore del flag scende
      | da 1 a 0 ricomincia ad integrare
      | dalla condizione iniziale che gli
      | sta arrivando in quel momento
  wB : Inport
  flag : Inport  Port=2
  IC_313 : Inport  Port=3
  Create DCM_BN_313 Matrix : MATLAB Function  TreatAsAtomicUnit=on
  Differential Equations 313 : Subsystem
  Integrator : Integrator  ExternalReset=falling  InitialConditionSource=external  InitialCondition=[phi_0; theta_0; psi_0]  WrapState=on
  DCM_BN_313 : Outport
  wires:
  wB/1 -> Differential Equations 313/1(wB)
  Differential Equations 313/1(EA_BN_313_der) -> Integrator/1
  Create DCM_BN_313 Matrix/1(DCM_BN_313) -> DCM_BN_313/1
  Integrator/1 -> Differential Equations 313/2(EA_BN_313), Create DCM_BN_313 Matrix/1(EA_BN_313)
  IC_313/1 -> Integrator/3
  flag/1 -> Integrator/2

== system Model/KINEMATICS/FinalConditions ==
  DCM : Inport
  Display : Display
  MATLAB Function : MATLAB Function  TreatAsAtomicUnit=on
  To Workspace : ToWorkspace  VariableName=simout5  SaveFormat=Timeseries  SampleTime=-1
  wires:
  MATLAB Function/1(Ang0) -> To Workspace/1, Display/1
  DCM/1 -> MATLAB Function/1(A0)

== system Model/SENSORS/Gyro ==
  w : Inport
  ARW : Subsystem
  Constant : Constant  Value=Aorthsens
  Cscalefactor1 : Subsystem
  Discrete-Time Integrator : DiscreteIntegrator  InitialCondition=[0;0;0]  SampleTime=-1  ICPrevOutput=DiscIntNeverNeededParam  ICPrevScaledInput=DiscIntNeverNeededParam
  Product : Product  Multiplication=Matrix(*)
  Product1 : Product  Multiplication=Matrix(*)
  RRW : Subsystem
  Sum : Sum  Inputs=+++
  w_gyro : Outport
  wires:
  Cscalefactor1/1(C) -> Product1/1
  Constant/1 -> Product/1
  Sum/1 -> w_gyro/1
  w/1 -> Cscalefactor1/1(w), Product/2
  ARW/1(Out1) -> Sum/2
  Discrete-Time Integrator/1 -> Sum/3
  RRW/1(Out1) -> Discrete-Time Integrator/1
  Product/1 -> Product1/2
  Product1/1 -> Sum/1

== system Model/SENSORS/StarCat ==
  Abn : Inport
  Constant : Constant  Value=starcat
  Error : Subsystem
  MATLAB Function : MATLAB Function  TreatAsAtomicUnit=on
  Product : Product  Multiplication=Matrix(*)
  Product1 : Product  Multiplication=Matrix(*)
  Pseudoinverse : dspinverses/Pseudoinverse  wanterr=off  SimulateUsing=Interpreted execution
      settings: SourceProductBaseCode=DS
  rPolarisN : Subsystem
  StarSensor : Outport
  FlagStars : Outport  Port=2
  wires:
  Constant/1 -> rPolarisN/1(Ra,Dec)
  rPolarisN/1(rn) -> MATLAB Function/1(catrn)
  Abn/1 -> Product/1, MATLAB Function/2(Abn)
  MATLAB Function/1(Vn) -> Pseudoinverse/1, Product/2  "Vn"
  Product/1 -> Error/1(Sreal)  "Sb"
  Error/1(Ssens) -> Product1/1
  Pseudoinverse/1 -> Product1/2
  Product1/1 -> StarSensor/1
  MATLAB Function/2(num) -> FlagStars/1

== system Model/ACTUATORS/RW/Mapping actuator ==
  Uideal : Inport
  w_gyro : Inport  Port=2
  Configuration : Inport  Port=3
  Cross Product : matrix_library/Cross Product
      settings: SourceProductBaseCode=SL
  Discrete-Time Integrator : DiscreteIntegrator  InitialCondition=[0;0;0;0]  SampleTime=-1  ICPrevOutput=DiscIntNeverNeededParam  ICPrevScaledInput=DiscIntNeverNeededParam
  Gain : Gain  Gain=-1
  Product : Product  Multiplication=Matrix(*)
  Product1 : Product  Multiplication=Matrix(*)
  Pseudoinverse : dspinverses/Pseudoinverse  wanterr=off  SimulateUsing=Interpreted execution
      settings: SourceProductBaseCode=DS
  Sum : Sum
  ElectricMotor : Outport
  wires:
  Gain/1 -> Product/1
  Configuration/1 -> Product1/1, Pseudoinverse/1
  Cross Product/1 -> Sum/2  "w ^ Ahr"
  Discrete-Time Integrator/1 -> Product1/2  "hr"
  Product/1 -> ElectricMotor/1, Discrete-Time Integrator/1
  Pseudoinverse/1 -> Gain/1
  Sum/1 -> Product/2  "Mc+w^Ahr"
  Product1/1 -> Cross Product/2  "A*hr"
  Uideal/1 -> Sum/1
  w_gyro/1 -> Cross Product/1

== system Model/ACTUATORS/RW/RealRW ==
  Configuration : Inport
  w_real : Inport  Port=2
  Mr : Inport  Port=3
  Cross Product : matrix_library/Cross Product
      settings: SourceProductBaseCode=SL
  Desat : Subsystem
  Discrete-Time Integrator : DiscreteIntegrator  InitialCondition=hr0  SampleTime=-1  ICPrevOutput=DiscIntNeverNeededParam  ICPrevScaledInput=DiscIntNeverNeededParam
  Product : Product  Multiplication=Matrix(*)
  Product1 : Product  Multiplication=Matrix(*)
  Saturation : Saturate  UpperLimit=maxT  LowerLimit=-maxT
  Sum : Sum  Inputs=--
  Switch : Switch  Criteria=u2 > Threshold
  To Workspace : ToWorkspace  VariableName=simout2  SaveFormat=Timeseries  SampleTime=-1
  Zero-Order Hold : ZeroOrderHold  SampleTime=1/fgyro
  Ureal : Outport
  FlagDesat : Outport  Port=2
  wires:
  Sum/1 -> Ureal/1
  Configuration/1 -> Product1/1, Product/1
  Product/1 -> Sum/1  "A*hr dot"
  Discrete-Time Integrator/1 -> To Workspace/1, Desat/1(Hr), Product1/2  "hr"
  w_real/1 -> Zero-Order Hold/1
  Product1/1 -> Cross Product/2  "Ahr"
  Cross Product/1 -> Sum/2  "w^Ahr"
  Switch/1 -> Discrete-Time Integrator/1, Product/2  "Mc=hr dot"
  Mr/1 -> Saturation/1
  Desat/2(Mmotorsat) -> Switch/1
  Desat/1(FlagDesat) -> FlagDesat/1, Switch/2
  Saturation/1 -> Switch/3
  Zero-Order Hold/1 -> Cross Product/1

== system Model/ACTUATORS/Thruster/On//Off logic ==
  Fideal : Inport
  Constant1 : Constant  Value=0
  Constant2 : Constant  Value=Fmax
  Constant3 : Constant  Value=[Fmax;Fmax;Fmax;Fmax]
  Demux : Demux
  GreaterThan : RelationalOperator  Operator=>  OutDataTypeStr=boolean  RndMeth=Simplest
  Mux : Mux
  Switch{,1..3} (4 alike) : Switch  Criteria=u2 > Threshold
  Freal : Outport
  wires:
  Switch2/1 -> Mux/3
  Constant1/1 -> Switch3/3, Switch2/3, Switch1/3, Switch/3
  Demux/3 -> Switch2/2
  Constant2/1 -> Switch3/1, Switch2/1, Switch1/1, Switch/1
  Switch/1 -> Mux/1
  Demux/4 -> Switch3/2
  Switch3/1 -> Mux/4
  Demux/1 -> Switch/2
  Demux/2 -> Switch1/2
  Switch1/1 -> Mux/2
  GreaterThan/1 -> Demux/1
  Constant3/1 -> GreaterThan/2
  Mux/1 -> Freal/1
  Fideal/1 -> GreaterThan/1

== system Model/ATTITUDE DETERMINATION ALGORITHMS/Kinematics with update from Star Tracker1/312 Euler Angles ==
  note: Quando il valore del flag
      | sale da 0 a 1 ricomincia
      | ad integrare dalla condizione
      | iniziale che gli sta arrivando
      | in quel momento
  IC_312 : Inport
  flag : Inport  Port=2
  wB : Inport  Port=3
  Create DCM_BN_312 Matrix : MATLAB Function  TreatAsAtomicUnit=on
  Differential Equations 312 : Subsystem
  Discrete-Time Integrator : DiscreteIntegrator  ExternalReset=either  InitialConditionSource=external  SampleTime=-1  ICPrevOutput=DiscIntNeverNeededParam  ICPrevScaledInput=DiscIntNeverNeededParam
  DCM_BN_312 : Outport
  wires:
  flag/1 -> Discrete-Time Integrator/2
  IC_312/1 -> Discrete-Time Integrator/3
  Discrete-Time Integrator/1 -> Differential Equations 312/2(EA_BN_312), Create DCM_BN_312 Matrix/1(EA_BN_312)
  Create DCM_BN_312 Matrix/1(DCM_BN_312) -> DCM_BN_312/1
  Differential Equations 312/1(EA_BN_312_der) -> Discrete-Time Integrator/1
  wB/1 -> Differential Equations 312/1(wB)

== system Model/ATTITUDE DETERMINATION ALGORITHMS/Kinematics with update from Star Tracker1/313 Euler Angles ==
  note: Quando il valore del flag scende
      | da 1 a 0 ricomincia ad integrare
      | dalla condizione iniziale che gli
      | sta arrivando in quel momento
  wB : Inport
  flag : Inport  Port=2
  IC_313 : Inport  Port=3
  Create DCM_BN_313 Matrix : MATLAB Function  TreatAsAtomicUnit=on
  Differential Equations 313 : Subsystem
  Discrete-Time Integrator : DiscreteIntegrator  ExternalReset=either  InitialConditionSource=external  SampleTime=-1  ICPrevOutput=DiscIntNeverNeededParam  ICPrevScaledInput=DiscIntNeverNeededParam
  DCM_BN_313 : Outport
  wires:
  flag/1 -> Discrete-Time Integrator/2
  IC_313/1 -> Discrete-Time Integrator/3
  Discrete-Time Integrator/1 -> Create DCM_BN_313 Matrix/1(EA_BN_313), Differential Equations 313/2(EA_BN_313)
  Create DCM_BN_313 Matrix/1(DCM_BN_313) -> DCM_BN_313/1
  Differential Equations 313/1(EA_BN_313_der) -> Discrete-Time Integrator/1
  wB/1 -> Differential Equations 313/1(wB)

== system Model/ATTITUDE DETERMINATION ALGORITHMS/SwitchAttitudeDetermination/SunPositionRespectN ==
  Digital Clock : DigitalClock  SampleTime=1/fgyro
  MATLAB Function : MATLAB Function  TreatAsAtomicUnit=on
  Normalize Vector : vrlib/Utilities/Normalize Vector  maxzero=0
  Rs : Constant  Value=148390000
  eps : Constant  Value=23.45
  n_sun : Constant  Value=2*pi/31536000
  sn : Outport
  wires:
  eps/1 -> MATLAB Function/1(eps)
  n_sun/1 -> MATLAB Function/2(n_sun)
  Rs/1 -> MATLAB Function/3(Rs)
  Digital Clock/1 -> MATLAB Function/4(time)
  MATLAB Function/1(sn) -> Normalize Vector/1
  Normalize Vector/1 -> sn/1

== system Model/CONTROL ALGORITHMS/Tracking/Subsystem ==
  Abn : Inport
  Aln : Inport  Port=2
  Product : Product  Multiplication=Matrix(*)
  Transpose : matrix_library/Transpose
      settings: SourceProductBaseCode=SL
  Ae : Outport
  wires:
  Abn/1 -> Product/1
  Aln/1 -> Transpose/1
  Transpose/1 -> Product/2
  Product/1 -> Ae/1  "Ae"

== system Model/CONTROL ALGORITHMS/Tracking/we ==
  Ae : Inport
  wd : Inport  Port=2
  wgyro : Inport  Port=3
  Product : Product  Multiplication=Matrix(*)
  Sum : Sum  Inputs=+-
  we : Outport
  wires:
  Product/1 -> Sum/2
  Sum/1 -> we/1
  Ae/1 -> Product/1
  wgyro/1 -> Sum/1
  wd/1 -> Product/2

== system Model/ENVIRONMENT DISTURBANCE TORQUES/OrbitRadialDirection/Subsystem ==
  Theta : Inport
  e : Inport  Port=2
  a : Inport  Port=3
  Constant : Constant
  Cos : Trigonometry  Operator=cos
  Divide : Product  Inputs=/*
  Product : Product
  Product1 : Product
  Square : Math  Operator=square  SaturateOnIntegerOverflow=on
  Sum : Sum  Inputs=-+
  Sum1 : Sum
  R : Outport
  wires:
  Theta/1 -> Cos/1
  e/1 -> Product1/2, Square/1
  Square/1 -> Sum/1
  Constant/1 -> Sum1/2, Sum/2
  Sum/1 -> Product/1
  a/1 -> Product/2
  Cos/1 -> Product1/1
  Product1/1 -> Sum1/1
  Sum1/1 -> Divide/1
  Product/1 -> Divide/2
  Divide/1 -> R/1

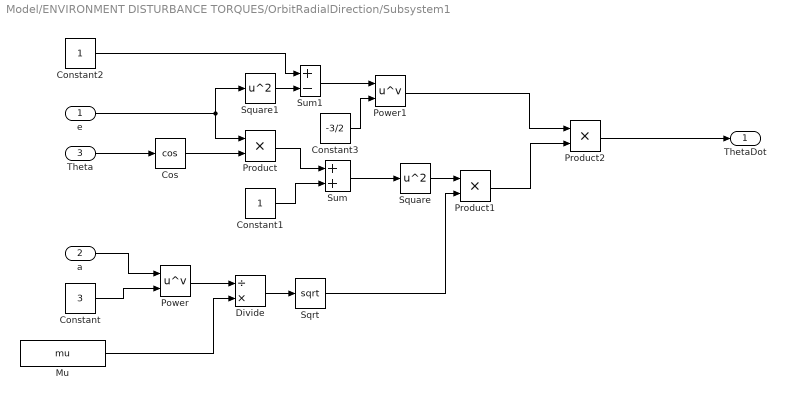
== system Model/ENVIRONMENT DISTURBANCE TORQUES/OrbitRadialDirection/Subsystem1 ==
  e : Inport
  a : Inport  Port=2
  Theta : Inport  Port=3
  Constant : Constant  Value=3
  Constant1 : Constant
  Constant2 : Constant
  Constant3 : Constant  Value=-3/2
  Cos : Trigonometry  Operator=cos
  Divide : Product  Inputs=/*
  Mu : Constant  Value=mu
  Power : Math  Operator=pow  SaturateOnIntegerOverflow=on
  Power1 : Math  Operator=pow  SaturateOnIntegerOverflow=on
  Product : Product
  Product1 : Product
  Product2 : Product
  Sqrt : Sqrt  SaturateOnIntegerOverflow=on
  Square : Math  Operator=square  SaturateOnIntegerOverflow=on
  Square1 : Math  Operator=square  SaturateOnIntegerOverflow=on
  Sum : Sum
  Sum1 : Sum  Inputs=+-
  ThetaDot : Outport
  wires:
  Constant/1 -> Power/2
  a/1 -> Power/1
  Power/1 -> Divide/1
  Mu/1 -> Divide/2
  Divide/1 -> Sqrt/1
  Theta/1 -> Cos/1
  Cos/1 -> Product/2
  e/1 -> Product/1, Square1/1
  Constant1/1 -> Sum/2
  Product/1 -> Sum/1
  Sum/1 -> Square/1
  Square/1 -> Product1/1
  Sqrt/1 -> Product1/2
  Square1/1 -> Sum1/2
  Constant2/1 -> Sum1/1
  Sum1/1 -> Power1/1
  Constant3/1 -> Power1/2
  Product1/1 -> Product2/2
  Power1/1 -> Product2/1
  Product2/1 -> ThetaDot/1
